simulink model "Actuator"  (R2025b)
settings: Solver=ode15s  StartTime=0.0  StopTime=100  RelTol=1e-6
settings Model: Creator=ikita  LastModifiedBy=mikol

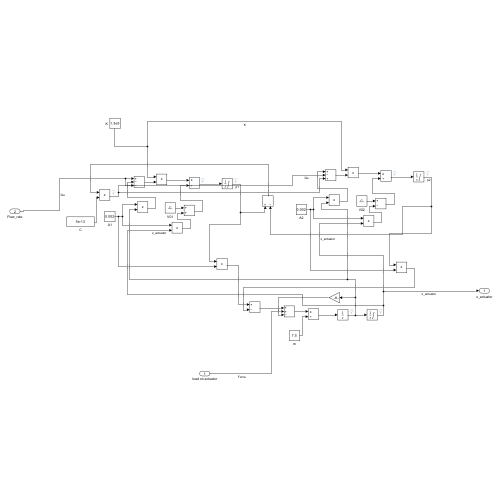
[thumbnail: Simulink's stored preview of the top-level diagram]
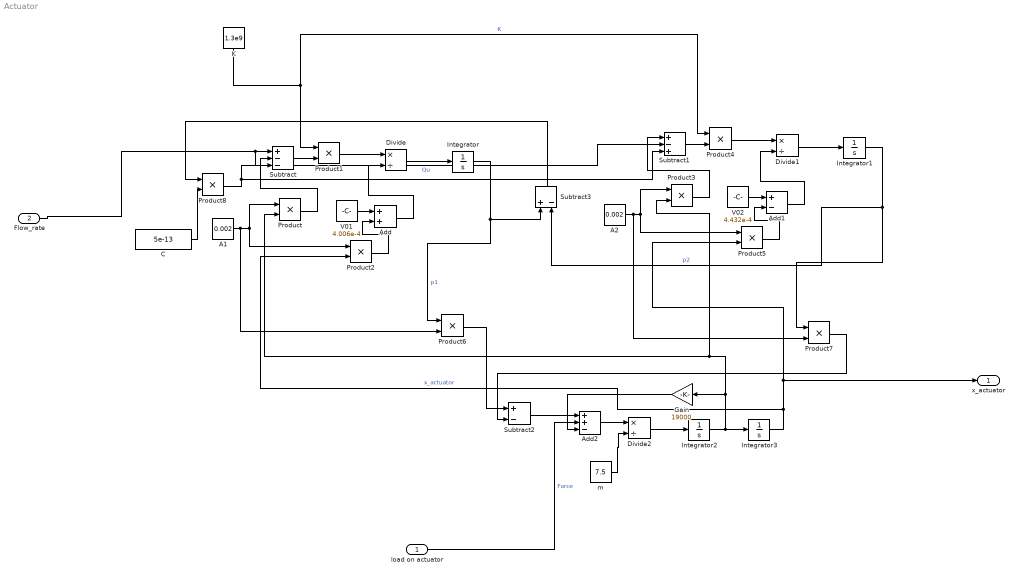
== system Actuator ==
  load on actuator : Inport
  Flow_rate : Inport  Port=2
  A1 : Constant  Value=0.002
  A2 : Constant  Value=0.002
  Add : Sum
  Add1 : Sum  Inputs=+-
  Add2 : Sum  Inputs=++-
  C : Constant  Value=5e-13
  Divide : Product  Inputs=*/
  Divide1 : Product  Inputs=*/
  Divide2 : Product  Inputs=*/
  Gain : Gain  Gain=19000
  Integrator : Integrator  InitialCondition=1e7  LimitOutput=on  LowerSaturationLimit=0
  Integrator1 : Integrator  InitialCondition=1e7  LimitOutput=on  LowerSaturationLimit=0
  Integrator2 : Integrator
  Integrator3 : Integrator  LimitOutput=on  UpperSaturationLimit=0.221  LowerSaturationLimit=-0.2
  K : Constant  Value=1.3e9
  Product{,1..8} (9 alike) : Product
  Subtract : Sum  Inputs=+--
  Subtract1 : Sum  Inputs=+-+
  Subtract2 : Sum  Inputs=+-
  Subtract3 : Sum  Inputs=+-
  V01 : Constant  Value=4.006e-4
  V02 : Constant  Value=4.432e-4
  m : Constant  Value=7.5
  x_actuator : Outport
  wires:
  Flow_rate/1 -> Subtract1/2, Subtract/1  "Qu"
  A1/1 -> Product6/2, Product/1, Product2/1
  Product/1 -> Subtract/2
  Subtract/1 -> Product1/2
  Product1/1 -> Divide/1
  Add/1 -> Divide/2
  V01/1 -> Add/1
  Product2/1 -> Add/2
  Divide/1 -> Integrator/1
  Integrator/1 -> Subtract3/1, Product6/1  "p1"
  Integrator1/1 -> Subtract3/2, Product7/1  "p2"
  Add1/1 -> Divide1/2
  Integrator2/1 -> Gain/1, Product3/2, Product/2, Integrator3/1
  Subtract1/1 -> Product4/2
  Product5/1 -> Add1/2
  Divide1/1 -> Integrator1/1
  A2/1 -> Product7/2, Product3/1, Product5/1
  V02/1 -> Add1/1
  Product3/1 -> Subtract1/1
  Product4/1 -> Divide1/1
  K/1 -> Product1/1, Product4/1  "K"
  Integrator3/1 -> Product2/2, x_actuator/1, Product5/2  "x_actuator"
  Product6/1 -> Subtract2/1
  Product7/1 -> Subtract2/2
  Subtract2/1 -> Add2/1
  load on actuator/1 -> Add2/2  "Force"
  Add2/1 -> Divide2/1
  m/1 -> Divide2/2
  Divide2/1 -> Integrator2/1
  Gain/1 -> Add2/3
  Product8/1 -> Subtract/3, Subtract1/3
  C/1 -> Product8/2
  Subtract3/1 -> Product8/1
